simulink model "third"  (R2016a)
settings: Solver=VariableStepAuto  StartTime=0.0  StopTime=10.0  RelTol=1e-3
settings Model: Creator=kypis  LastModifiedBy=kypis

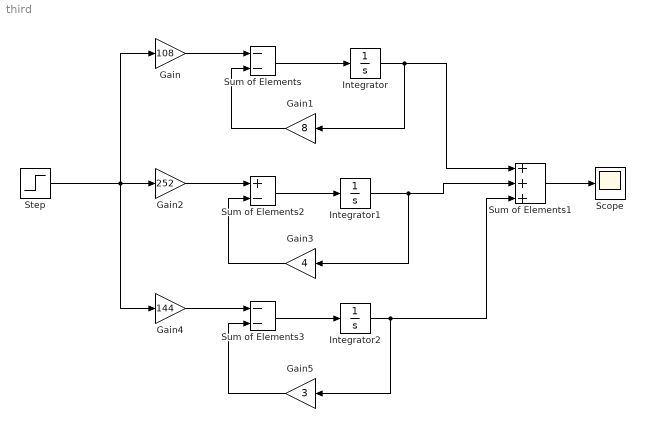
== system third ==
  Gain : Gain  Gain=108
  Gain1 : Gain  Gain=8
  Gain2 : Gain  Gain=252
  Gain3 : Gain  Gain=4
  Gain4 : Gain  Gain=144
  Gain5 : Gain  Gain=3
  Integrator : Integrator
  Integrator1 : Integrator
  Integrator2 : Integrator
  Scope : Scope
  Step : Step  Time=0  SampleTime=0
  Sum of Elements : Sum  Inputs=--
  Sum of Elements1 : Sum  Inputs=+++
  Sum of Elements2 : Sum  Inputs=+-
  Sum of Elements3 : Sum  Inputs=--
  wires:
  Step/1 -> Gain4/1, Gain/1, Gain2/1
  Gain/1 -> Sum of Elements/1
  Sum of Elements/1 -> Integrator/1
  Integrator/1 -> Gain1/1, Sum of Elements1/1
  Gain1/1 -> Sum of Elements/2
  Gain2/1 -> Sum of Elements2/1
  Sum of Elements2/1 -> Integrator1/1
  Integrator1/1 -> Gain3/1, Sum of Elements1/2
  Gain3/1 -> Sum of Elements2/2
  Gain4/1 -> Sum of Elements3/1
  Sum of Elements3/1 -> Integrator2/1
  Integrator2/1 -> Gain5/1, Sum of Elements1/3
  Gain5/1 -> Sum of Elements3/2
  Sum of Elements1/1 -> Scope/1
